simulink model "untitled"  (R2021a)
settings: Solver=VariableStepAuto  StartTime=0.0  StopTime=20000  RelTol=1e-3
values from neighbouring files (symbols this model uses):
  dtheta_GMO = sqrt(muy/r_GMO^3)    [Parameters.m]    (also in Spacecraft_Attitude_States.m)
  dtheta_LMO = sqrt(muy/r_LMO^3)    [Parameters.m]    (also in Spacecraft_Attitude_States.m)
  I = [10 0 0;0 5 0;0 0 7.5]    [Parameters.m]    (also in Spacecraft_Attitude_States.m)
  i0_GMO = 0    [Parameters.m]    (also in Spacecraft_Attitude_States.m)
  i0_LMO = pi/6    (= 0.523598775598)    [Parameters.m]    (also in Spacecraft_Attitude_States.m)
  K = 5    [Parameters.m]    (also in Spacecraft_Attitude_States.m)
  Omega0_GMO = 0    [Parameters.m]    (also in Spacecraft_Attitude_States.m)
  Omega0_LMO = pi/9    (= 0.349065850399)    [Parameters.m]    (also in Spacecraft_Attitude_States.m)
  P = 10*eye(3)    [Parameters.m]    (also in Spacecraft_Attitude_States.m)
  r_GMO = 20424.2*10^3    (= 20424200)    [Parameters.m]    (also in Spacecraft_Attitude_States.m = 20424.2)
  r_LMO = R + h    (= 3796190)    [Parameters.m]    (also in Spacecraft_Attitude_States.m = 3796.19)
  T1 = 800    [Parameters.m]
  T2 = 2500    [Parameters.m]
  theta0_GMO = 250*pi/180    (= 4.36332312999)    [Parameters.m]    (also in Spacecraft_Attitude_States.m)
  theta0_LMO = pi/3    (= 1.0471975512)    [Parameters.m]    (also in Spacecraft_Attitude_States.m)
libraries: sharedtransform x1
settings Model: Creator=VTX  LastModifiedBy=VTX

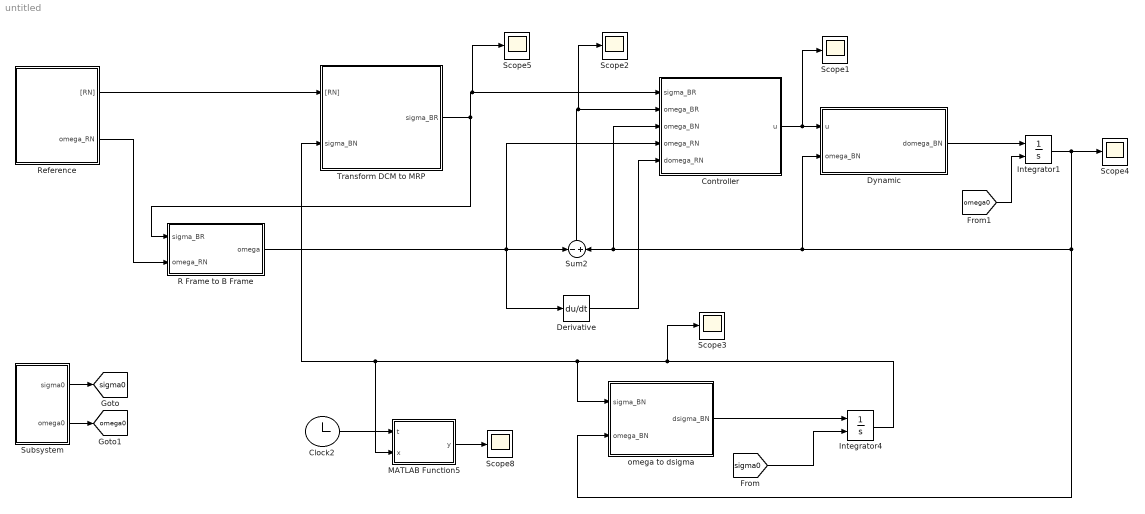
== system untitled ==
  Clock2 : Clock
  Controller : MATLAB Function  TreatAsAtomicUnit=on
  Derivative : Derivative
  Dynamic : MATLAB Function  TreatAsAtomicUnit=on
  Integrator1 : Integrator  InitialConditionSource=external  InitialCondition=[1;1.75;-2.2]*pi/180
  Integrator4 : Integrator  InitialConditionSource=external  InitialCondition=[0.3;-0.4;0.5]
  MATLAB Function5 : MATLAB Function  TreatAsAtomicUnit=on
  R Frame to B Frame : MATLAB Function  TreatAsAtomicUnit=on
  Reference : Subsystem
  Scope{1..5,8} (6 alike) : Scope
  Subsystem : Subsystem
  Sum2 : Sum  Inputs=-|+
  Transform DCM to MRP : Subsystem
  omega to dsigma : MATLAB Function  TreatAsAtomicUnit=on
  tag scope: omega0=global, sigma0=global
  wires:
  Integrator1/1 -> Dynamic/2(omega_BN), Controller/3(omega_BN), Sum2/2, omega to dsigma/2(omega_BN), Scope4/1
  Sum2/1 -> Scope2/1, Controller/2(omega_BR)
  [sigma0] -> Integrator4/2
  [omega0] -> Integrator1/2
  Derivative/1 -> Controller/5(domega_RN)
  Clock2/1 -> MATLAB Function5/1(t)
  Integrator4/1 -> Scope3/1, Transform DCM to MRP/2(sigma_BN), MATLAB Function5/2(x), omega to dsigma/1(sigma_BN)
  Subsystem/1(sigma0) -> [sigma0]
  Subsystem/2(omega0) -> [omega0]
  Dynamic/1(domega_BN) -> Integrator1/1
  Reference/1("[RN]") -> Transform DCM to MRP/1("[RN]")
  Transform DCM to MRP/1(sigma_BR) -> R Frame to B Frame/1(sigma_BR), Scope5/1, Controller/1(sigma_BR)
  R Frame to B Frame/1(omega) -> Sum2/1, Derivative/1, Controller/4(omega_RN)
  omega to dsigma/1(dsigma_BN) -> Integrator4/1
  Controller/1(u) -> Scope1/1, Dynamic/1(u)
  Reference/2(omega_RN) -> R Frame to B Frame/2(omega_RN)
  MATLAB Function5/1(y) -> Scope8/1

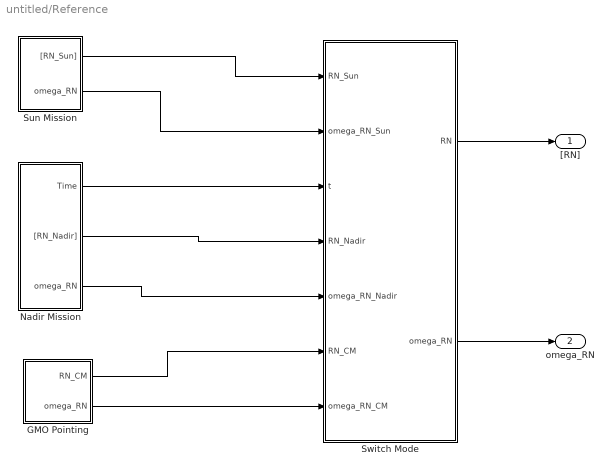
== system untitled/Reference ==
  GMO Pointing : Subsystem
  Nadir Mission : Subsystem
  Sun Mission : Subsystem
  Switch Mode : MATLAB Function  TreatAsAtomicUnit=on
  "[RN]" : Outport
  omega_RN : Outport  Port=2
  wires:
  Switch Mode/2(omega_RN) -> omega_RN/1
  Switch Mode/1(RN) -> "[RN]"/1
  Sun Mission/1("[RN_Sun]") -> Switch Mode/1(RN_Sun)
  Sun Mission/2(omega_RN) -> Switch Mode/2(omega_RN_Sun)
  Nadir Mission/1(Time) -> Switch Mode/3(t)
  Nadir Mission/2("[RN_Nadir]") -> Switch Mode/4(RN_Nadir)
  Nadir Mission/3(omega_RN) -> Switch Mode/5(omega_RN_Nadir)
  GMO Pointing/1(RN_CM) -> Switch Mode/6(RN_CM)
  GMO Pointing/2(omega_RN) -> Switch Mode/7(omega_RN_CM)

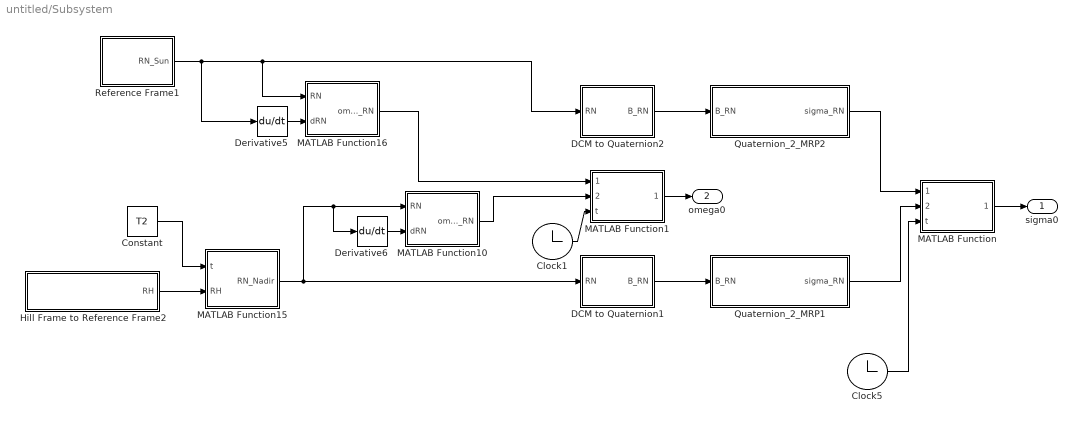
== system untitled/Subsystem ==
  Clock1 : Clock
  Clock5 : Clock
  Constant : Constant  Value=T2
  DCM to Quaternion1 : MATLAB Function  TreatAsAtomicUnit=on
  DCM to Quaternion2 : MATLAB Function  TreatAsAtomicUnit=on
  Derivative5 : Derivative
  Derivative6 : Derivative
  Hill Frame to Reference Frame2 : MATLAB Function  TreatAsAtomicUnit=on
  MATLAB Function : MATLAB Function  TreatAsAtomicUnit=on
  MATLAB Function1 : MATLAB Function  TreatAsAtomicUnit=on
  MATLAB Function10 : MATLAB Function  TreatAsAtomicUnit=on
  MATLAB Function15 : MATLAB Function  TreatAsAtomicUnit=on
  MATLAB Function16 : MATLAB Function  TreatAsAtomicUnit=on
  Quaternion_2_MRP1 : MATLAB Function  TreatAsAtomicUnit=on
  Quaternion_2_MRP2 : MATLAB Function  TreatAsAtomicUnit=on
  Reference Frame1 : MATLAB Function  TreatAsAtomicUnit=on
  sigma0 : Outport
  omega0 : Outport  Port=2
  wires:
  MATLAB Function15/1(RN_Nadir) -> DCM to Quaternion1/1(RN), Derivative6/1, MATLAB Function10/1(RN)
  Reference Frame1/1(RN_Sun) -> Derivative5/1, DCM to Quaternion2/1(RN), MATLAB Function16/1(RN)
  ? -> ?
  Hill Frame to Reference Frame2/1(RH) -> MATLAB Function15/2(RH)
  Derivative5/1 -> MATLAB Function16/2(dRN)
  MATLAB Function16/1(omega_RN) -> MATLAB Function1/1(omega_RN_Sun)
  Derivative6/1 -> MATLAB Function10/2(dRN)
  Constant/1 -> MATLAB Function15/1(t)
  DCM to Quaternion2/1(B_RN) -> Quaternion_2_MRP2/1(B_RN)
  DCM to Quaternion1/1(B_RN) -> Quaternion_2_MRP1/1(B_RN)
  Quaternion_2_MRP2/1(sigma_RN) -> MATLAB Function/1(sigma_RN_Sun)
  Quaternion_2_MRP1/1(sigma_RN) -> MATLAB Function/2(sigma_RN_Nadir)
  Clock5/1 -> MATLAB Function/3(t)
  MATLAB Function/1(sigma0) -> sigma0/1
  MATLAB Function10/1(omega_RN) -> MATLAB Function1/2(omega_RN_Nadir)
  Clock1/1 -> MATLAB Function1/3(t)
  MATLAB Function1/1(omega0) -> omega0/1

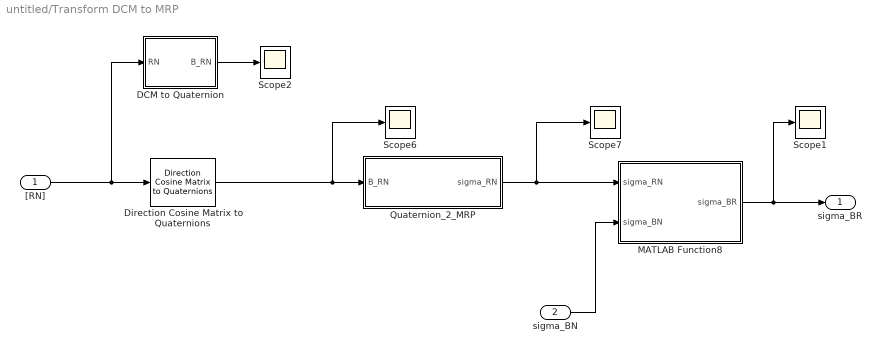
== system untitled/Transform DCM to MRP ==
  "[RN]" : Inport
  sigma_BN : Inport  Port=2
  DCM to Quaternion : MATLAB Function  TreatAsAtomicUnit=on
  Direction Cosine Matrix to Quaternions : sharedtransform/Direction Cosine Matrix  to Quaternions  aMode=0  action=None  tolerance=eps(2)
      settings: SourceProductBaseCode=AE,PW,DR,MT,UV,VE
  MATLAB Function8 : MATLAB Function  TreatAsAtomicUnit=on
  Quaternion_2_MRP : MATLAB Function  TreatAsAtomicUnit=on
  Scope{1..2,6..7} (4 alike) : Scope
  sigma_BR : Outport
  wires:
  Direction Cosine Matrix to Quaternions/1 -> Scope6/1, Quaternion_2_MRP/1(B_RN)
  Quaternion_2_MRP/1(sigma_RN) -> Scope7/1, MATLAB Function8/1(sigma_RN)
  sigma_BN/1 -> MATLAB Function8/2(sigma_BN)
  MATLAB Function8/1(sigma_BR) -> Scope1/1, sigma_BR/1
  "[RN]"/1 -> DCM to Quaternion/1(RN), Direction Cosine Matrix to Quaternions/1
  DCM to Quaternion/1(B_RN) -> Scope2/1

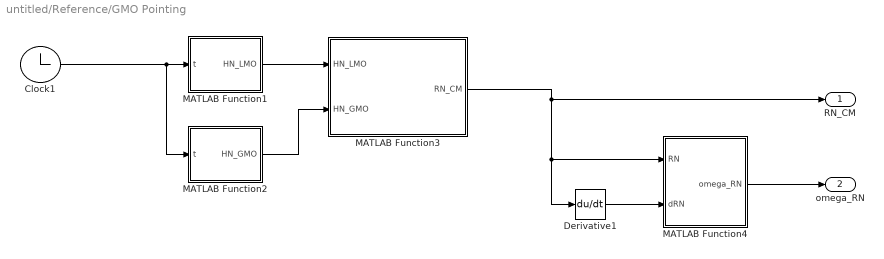
== system untitled/Reference/GMO Pointing ==
  Clock1 : Clock
  Derivative1 : Derivative
  MATLAB Function1 : MATLAB Function  TreatAsAtomicUnit=on
  MATLAB Function2 : MATLAB Function  TreatAsAtomicUnit=on
  MATLAB Function3 : MATLAB Function  TreatAsAtomicUnit=on
  MATLAB Function4 : MATLAB Function  TreatAsAtomicUnit=on
  RN_CM : Outport
  omega_RN : Outport  Port=2
  wires:
  Derivative1/1 -> MATLAB Function4/2(dRN)
  MATLAB Function1/1(HN_LMO) -> MATLAB Function3/1(HN_LMO)
  Clock1/1 -> MATLAB Function2/1(t), MATLAB Function1/1(t)
  MATLAB Function2/1(HN_GMO) -> MATLAB Function3/2(HN_GMO)
  MATLAB Function3/1(RN_CM) -> Derivative1/1, MATLAB Function4/1(RN), RN_CM/1
  MATLAB Function4/1(omega_RN) -> omega_RN/1

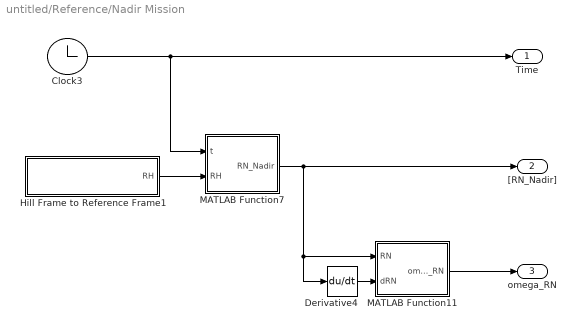
== system untitled/Reference/Nadir Mission ==
  Clock3 : Clock
  Derivative4 : Derivative
  Hill Frame to Reference Frame1 : MATLAB Function  TreatAsAtomicUnit=on
  MATLAB Function11 : MATLAB Function  TreatAsAtomicUnit=on
  MATLAB Function7 : MATLAB Function  TreatAsAtomicUnit=on
  Time : Outport
  "[RN_Nadir]" : Outport  Port=2
  omega_RN : Outport  Port=3
  wires:
  Clock3/1 -> Time/1, MATLAB Function7/1(t)
  MATLAB Function11/1(omega_RN) -> omega_RN/1
  MATLAB Function7/1(RN_Nadir) -> "[RN_Nadir]"/1, Derivative4/1, MATLAB Function11/1(RN)
  Hill Frame to Reference Frame1/1(RH) -> MATLAB Function7/2(RH)
  Derivative4/1 -> MATLAB Function11/2(dRN)

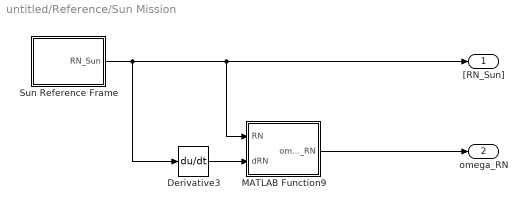
== system untitled/Reference/Sun Mission ==
  Derivative3 : Derivative
  MATLAB Function9 : MATLAB Function  TreatAsAtomicUnit=on
  Sun Reference Frame : MATLAB Function  TreatAsAtomicUnit=on
  "[RN_Sun]" : Outport
  omega_RN : Outport  Port=2
  wires:
  Derivative3/1 -> MATLAB Function9/2(dRN)
  Sun Reference Frame/1(RN_Sun) -> Derivative3/1, "[RN_Sun]"/1, MATLAB Function9/1(RN)
  MATLAB Function9/1(omega_RN) -> omega_RN/1

== matlab function untitled/Reference/GMO Pointing/MATLAB Function3 ==
  data: RN_CM output; HN_LMO input; HN_GMO input; r_LMO parameter; r_GMO parameter
function RN_CM = fcn(HN_LMO, HN_GMO,r_LMO, r_GMO)
    R_LMO = r_LMO*HN_LMO'*[1 0 0]';
    R_GMO = r_GMO*HN_GMO'*[1 0 0]';
    delta_R = R_GMO - R_LMO;
    
    r1 = delta_R/norm(delta_R);
    r2 = cross(delta_R,[0 0 1]')/norm(cross(delta_R,[0 0 1]'));
    r3 = cross(r1,r2);
    
    RN_CM = [r1 r2 r3]';
end

== matlab function untitled/Reference/GMO Pointing/MATLAB Function4 ==
  data: RN input; omega_RN output; dRN input
function omega_RN = fcn(RN,dRN)
    omega_RN_tidle = -dRN*RN';
    o1 = omega_RN_tidle(3,2);
    o2 = omega_RN_tidle(1,3);
    o3 = omega_RN_tidle(2,1);
    omega_RN = [o1 o2 o3]';
end

== matlab function untitled/MATLAB Function5 ==
  data: t input; y output; x input; T1 parameter
function y = fcn(t,x,T1)
    y = [0 0 0]';
    if t == T1
        y = x;
    end
end

== matlab function untitled/Subsystem/Hill Frame to Reference Frame2 ==
  data: RH output
function RH = fcn()
RH = [-1 0 0;0 1 0;0 0 -1];
end

== matlab function untitled/Subsystem/MATLAB Function10 ==
  data: RN input; omega_RN output; dRN input
function omega_RN = fcn(RN,dRN)
    omega_RN_tidle = -dRN*RN';
    o1 = omega_RN_tidle(3,2);
    o2 = omega_RN_tidle(1,3);
    o3 = omega_RN_tidle(2,1);
    omega_RN = [o1 o2 o3]';
end

== matlab function untitled/Subsystem/DCM to Quaternion2 ==
  data: RN input; B_RN output size=4
function B_RN = fcn(RN)
    trace = RN(1,1) + RN(2,2) + RN(3,3);
    beta0 = (0.25*(1 + trace));
    beta1 = (0.25*(1 + 2*RN(1,1) - trace));
    beta2 = (0.25*(1 + 2*RN(2,2) - trace));
    beta3 = (0.25*(1 + 2*RN(3,3) - trace));
    
    m = max([beta0 beta1 beta2 beta3]);

    B0 = 0; B1 = 0; B2 = 0; B3 = 0;
    
    if beta0 == m
        B0 = sqrt(beta0);
        B1 = (RN(2,3)-RN(3,2))/(4*B0);
        B2 = (RN(3,1)-RN(1,3))/(4*B0);
        B3 = (RN(1,2)-RN(2,1))/(4*B0);
    elseif beta1 == m
        B1 = sqrt(beta1);
        B0 = (RN(2,3)-RN(3,2))/(4*B1);
        B2 = (RN(1,2)+RN(2,1))/(4*B1);
        B3 = (RN(3,1)+RN(1,3))/(4*B1);
    elseif beta2 == m
        B2 = sqrt(beta2);
        B0 = (RN(3,1)-RN(1,3))/(4*B2);
        B1 = (RN(1,2)+RN(2,1))/(4*B2);
        B3 = (RN(2,3)+RN(3,2))/(4*B2);
    elseif beta3 == m
        B3 = sqrt(beta3);
        B0 = (RN(1,2)-RN(2,1))/(4*B3);
        B1 = (RN(3,1)+RN(1,3))/(4*B3);
        B2 = (RN(2,3)+RN(3,2))/(4*B3);
    end
    
    B_RN = [B0 B1 B2 B3]';
end

== matlab function untitled/Subsystem/Quaternion_2_MRP2 ==
  data: B_RN input; sigma_RN output
function sigma_RN  = fcn(B_RN)
    sigma1 = B_RN(2)/(1 + B_RN(1));
    sigma2 = B_RN(3)/(1 + B_RN(1));
    sigma3 = B_RN(4)/(1 + B_RN(1));
    
    sigma_RN = [sigma1 sigma2 sigma3]';

    if norm(sigma_RN) >= 1
        sigma1 = -B_RN(2)/(1 - B_RN(1));
        sigma2 = -B_RN(3)/(1 - B_RN(1));
        sigma3 = -B_RN(4)/(1 - B_RN(1));
    
        sigma_RN = [sigma1 sigma2 sigma3]';
    end   
end

== matlab function untitled/Subsystem/DCM to Quaternion1 ==
  data: RN input; B_RN output size=4
function B_RN = fcn(RN)
    trace = RN(1,1) + RN(2,2) + RN(3,3);
    beta0 = (0.25*(1 + trace));
    beta1 = (0.25*(1 + 2*RN(1,1) - trace));
    beta2 = (0.25*(1 + 2*RN(2,2) - trace));
    beta3 = (0.25*(1 + 2*RN(3,3) - trace));
    
    m = max([beta0 beta1 beta2 beta3]);

    B0 = 0; B1 = 0; B2 = 0; B3 = 0;
    
    if beta0 == m
        B0 = sqrt(beta0);
        B1 = (RN(2,3)-RN(3,2))/(4*B0);
        B2 = (RN(3,1)-RN(1,3))/(4*B0);
        B3 = (RN(1,2)-RN(2,1))/(4*B0);
    elseif beta1 == m
        B1 = sqrt(beta1);
        B0 = (RN(2,3)-RN(3,2))/(4*B1);
        B2 = (RN(1,2)+RN(2,1))/(4*B1);
        B3 = (RN(3,1)+RN(1,3))/(4*B1);
    elseif beta2 == m
        B2 = sqrt(beta2);
        B0 = (RN(3,1)-RN(1,3))/(4*B2);
        B1 = (RN(1,2)+RN(2,1))/(4*B2);
        B3 = (RN(2,3)+RN(3,2))/(4*B2);
    elseif beta3 == m
        B3 = sqrt(beta3);
        B0 = (RN(1,2)-RN(2,1))/(4*B3);
        B1 = (RN(3,1)+RN(1,3))/(4*B3);
        B2 = (RN(2,3)+RN(3,2))/(4*B3);
    end
    
    B_RN = [B0 B1 B2 B3]';
end

== matlab function untitled/Controller ==
  data: sigma_BR input; u output; omega_BR input; K parameter; P parameter; omega_BN input; omega_RN input; I parameter; domega_RN input
function u = fcn(sigma_BR,omega_BR,K,P,omega_BN,omega_RN, I,domega_RN)

    u = -K*sigma_BR - P*omega_BR;
    % u = -K*sigma_BR - P*omega_BR + I*(domega_RN - cross(omega_BN,omega_RN)) + cross(omega_BN,(I*omega_BN));
    
    u_max = 5;
    if abs(u) > u_max
        u = sign(u)*u_max;
    end
end

== matlab function untitled/Subsystem/MATLAB Function15 ==
  data: RN_Nadir output; t input; RH input; Omega0_LMO parameter; i0_LMO parameter; theta0_LMO parameter; dtheta_LMO parameter
function RN_Nadir  = fcn(t, RH,Omega0_LMO, i0_LMO, theta0_LMO, dtheta_LMO)
    %% Rotate about z axis
    Cz1 = [cos(Omega0_LMO) sin(Omega0_LMO) 0;-sin(Omega0_LMO) cos(Omega0_LMO) 0;0 0 1];

    %% Rotate about x axis
    Cx2 = [1 0 0;0 cos(i0_LMO) sin(i0_LMO);0 -sin(i0_LMO) cos(i0_LMO)];
    
    %% Rotate about z axis
    Cz3 = [cos(theta0_LMO + dtheta_LMO*t) sin(theta0_LMO + dtheta_LMO*t) 0;-sin(theta0_LMO + dtheta_LMO*t) cos(theta0_LMO + dtheta_LMO*t) 0;0 0 1];

    %% DCM from Inertial Frame to Hill Frame
    HN = Cz3*Cx2*Cz1;
    
    %% DCm from Inertial Frame to Reference Frame
    RN_Nadir = RH*HN;
end

== matlab function untitled/Subsystem/MATLAB Function16 ==
  data: RN input; omega_RN output; dRN input
function omega_RN = fcn(RN,dRN)
    omega_RN_tidle = -dRN*RN';
    o1 = omega_RN_tidle(3,2);
    o2 = omega_RN_tidle(1,3);
    o3 = omega_RN_tidle(2,1);
    omega_RN = [o1 o2 o3]';
end

== matlab function untitled/Subsystem/Quaternion_2_MRP1 ==
  data: B_RN input; sigma_RN output
function sigma_RN  = fcn(B_RN)
    sigma1 = B_RN(2)/(1 + B_RN(1));
    sigma2 = B_RN(3)/(1 + B_RN(1));
    sigma3 = B_RN(4)/(1 + B_RN(1));
    
    sigma_RN = [sigma1 sigma2 sigma3]';

    if norm(sigma_RN) >= 1
        sigma1 = -B_RN(2)/(1 - B_RN(1));
        sigma2 = -B_RN(3)/(1 - B_RN(1));
        sigma3 = -B_RN(4)/(1 - B_RN(1));
    
        sigma_RN = [sigma1 sigma2 sigma3]';
    end   
end

== matlab function untitled/Subsystem/Reference Frame1 ==
  data: RN_Sun output
function RN_Sun = fcn()
    RN_Sun = [-1 0 0;0 0 1;0 1 0];
end

== matlab function untitled/Subsystem/MATLAB Function ==
  data: sigma_RN_Sun input; sigma0 output; sigma_RN_Nadir input; t input; T1 parameter; T2 parameter
function sigma0 = fcn(sigma_RN_Sun,sigma_RN_Nadir,t,T1, T2)
    if t < T1
        sigma0 = [0.3;-0.4;0.5];
    elseif (t >= T1) && (t < T2)
        sigma0 = sigma_RN_Sun;
    else
        sigma0 = sigma_RN_Nadir;
    end
end

== matlab function untitled/Transform DCM to MRP/MATLAB Function8 ==
  data: sigma_BR output; sigma_RN input; sigma_BN input
function sigma_BR = fcn(sigma_RN, sigma_BN)
    sigma_BR = ((1 - norm(sigma_RN)^2)*sigma_BN - (1 - norm(sigma_BN)^2)*sigma_RN + 2*cross(sigma_BN,sigma_RN))/(1 + norm(sigma_RN)^2*norm(sigma_BN)^2 + 2*dot(sigma_RN,sigma_BN));
end

== matlab function untitled/Reference/Sun Mission/MATLAB Function9 ==
  data: RN input; omega_RN output; dRN input
function omega_RN = fcn(RN,dRN)
    omega_RN_tidle = -dRN*RN';
    o1 = omega_RN_tidle(3,2);
    o2 = omega_RN_tidle(1,3);
    o3 = omega_RN_tidle(2,1);
    omega_RN = [o1 o2 o3]';
end

== matlab function untitled/Transform DCM to MRP/Quaternion_2_MRP ==
  data: B_RN input; sigma_RN output
function sigma_RN  = fcn(B_RN)
    sigma1 = B_RN(2)/(1 + B_RN(1));
    sigma2 = B_RN(3)/(1 + B_RN(1));
    sigma3 = B_RN(4)/(1 + B_RN(1));
    
    sigma_RN = [sigma1 sigma2 sigma3]';

    if norm(sigma_RN) >= 1
        sigma1 = -B_RN(2)/(1 - B_RN(1));
        sigma2 = -B_RN(3)/(1 - B_RN(1));
        sigma3 = -B_RN(4)/(1 - B_RN(1));
    
        sigma_RN = [sigma1 sigma2 sigma3]';
    end   
end

== matlab function untitled/Reference/Sun Mission/Sun Reference Frame ==
  data: RN_Sun output
function RN_Sun = fcn()
    RN_Sun = [-1 0 0;0 0 1;0 1 0];
end

== matlab function untitled/Reference/Switch Mode ==
  data: RN_Sun input; omega_RN_Sun input; t input; RN_Nadir input; omega_RN_Nadir input; RN output; omega_RN output; RN_CM input; omega_RN_CM input; T1 parameter; T2 parameter
function [RN,omega_RN] = fcn(RN_Sun,omega_RN_Sun, t, RN_Nadir,omega_RN_Nadir,RN_CM,omega_RN_CM,T1, T2)
    RN = RN_Sun;
    omega_RN = omega_RN_Sun;
    if t > T1 && t <= T2
        RN = RN_Nadir;
        omega_RN = omega_RN_Nadir;
    elseif t > T2
        RN = RN_CM;
        omega_RN = omega_RN_CM;
    end
end

== matlab function untitled/omega to dsigma ==
  data: sigma_BN input; dsigma_BN output size=3; omega_BN input
function dsigma_BN = fcn(sigma_BN,omega_BN)
   sigma_tilde = [0 -sigma_BN(3) sigma_BN(2);sigma_BN(3) 0 -sigma_BN(1);-sigma_BN(2) sigma_BN(1) 0];
   dsigma_BN = 1/4*((1 - dot(sigma_BN,sigma_BN))*eye(3) + 2*sigma_tilde + 2*sigma_BN*sigma_BN')*omega_BN;
end

== matlab function untitled/Subsystem/MATLAB Function1 ==
  data: omega_RN_Sun input; omega0 output; omega_RN_Nadir input; t input; T1 parameter; T2 parameter
function omega0 = fcn(omega_RN_Sun,omega_RN_Nadir,t,T1, T2)
    if t < T1
        omega0 = [1;1.75;-2.2]*pi/180;
    elseif (t >= T1) && (t < T2)
        omega0 = omega_RN_Sun;
    else
        omega0 = omega_RN_Nadir;
    end
end

== matlab function untitled/Transform DCM to MRP/DCM to Quaternion ==
  data: RN input; B_RN output size=4
function B_RN = fcn(RN)
    trace = RN(1,1) + RN(2,2) + RN(3,3);
    beta0 = (0.25*(1 + trace));
    beta1 = (0.25*(1 + 2*RN(1,1) - trace));
    beta2 = (0.25*(1 + 2*RN(2,2) - trace));
    beta3 = (0.25*(1 + 2*RN(3,3) - trace));
    
    m = max([beta0 beta1 beta2 beta3]);

    B0 = 0; B1 = 0; B2 = 0; B3 = 0;
    
    if beta0 == m
        B0 = sqrt(beta0);
        B1 = (RN(2,3)-RN(3,2))/(4*B0);
        B2 = (RN(3,1)-RN(1,3))/(4*B0);
        B3 = (RN(1,2)-RN(2,1))/(4*B0);
    elseif beta1 == m
        B1 = sqrt(beta1);
        B0 = (RN(2,3)-RN(3,2))/(4*B1);
        B2 = (RN(1,2)+RN(2,1))/(4*B1);
        B3 = (RN(3,1)+RN(1,3))/(4*B1);
    elseif beta2 == m
        B2 = sqrt(beta2);
        B0 = (RN(3,1)-RN(1,3))/(4*B2);
        B1 = (RN(1,2)+RN(2,1))/(4*B2);
        B3 = (RN(2,3)+RN(3,2))/(4*B2);
    elseif beta3 == m
        B3 = sqrt(beta3);
        B0 = (RN(1,2)-RN(2,1))/(4*B3);
        B1 = (RN(3,1)+RN(1,3))/(4*B3);
        B2 = (RN(2,3)+RN(3,2))/(4*B3);
    end
    
    B_RN = [B0 B1 B2 B3]';
end

== matlab function untitled/Dynamic ==
  data: u input; domega_BN output size=3; omega_BN input; I parameter
function domega_BN = fcn(u,omega_BN, I)
    domega_BN = inv(I)*(cross(omega_BN,(I*omega_BN)) + u);
end

== matlab function untitled/Reference/Nadir Mission/Hill Frame to Reference Frame1 ==
  data: RH output
function RH = fcn()
RH = [-1 0 0;0 1 0;0 0 -1];
end

== matlab function untitled/R Frame to B Frame ==
  data: omega output; sigma_BR input; omega_RN input
function omega = fcn(sigma_BR, omega_RN)
    %% This function returns a DCM that is transformed from MRP
    s1 = sigma_BR(1);
    s2 = sigma_BR(2);
    s3 = sigma_BR(3);
    
    sigma_cross = [0 -s3 s2;s3 0 -s1;-s2 s1 0];
    
    DCM = eye(3) + (8*sigma_cross*sigma_cross - 4*(1 - dot(sigma_BR,sigma_BR))*sigma_cross)/(1 + dot(sigma_BR,sigma_BR))^2;
    
    omega  = DCM*omega_RN;
end

== matlab function untitled/Reference/Nadir Mission/MATLAB Function11 ==
  data: RN input; omega_RN output; dRN input
function omega_RN = fcn(RN,dRN)
    omega_RN_tidle = -dRN*RN';
    o1 = omega_RN_tidle(3,2);
    o2 = omega_RN_tidle(1,3);
    o3 = omega_RN_tidle(2,1);
    omega_RN = [o1 o2 o3]';
end

== matlab function untitled/Reference/GMO Pointing/MATLAB Function1 ==
  data: t input; HN_LMO output; Omega0_LMO parameter; i0_LMO parameter; theta0_LMO parameter; dtheta_LMO parameter
function HN_LMO  = fcn(t,Omega0_LMO, i0_LMO, theta0_LMO, dtheta_LMO)
    %% Rotate about z axis
    Cz1 = [cos(Omega0_LMO) sin(Omega0_LMO) 0;-sin(Omega0_LMO) cos(Omega0_LMO) 0;0 0 1];

    %% Rotate about x axis
    Cx2 = [1 0 0;0 cos(i0_LMO) sin(i0_LMO);0 -sin(i0_LMO) cos(i0_LMO)];
    
    %% Rotate about z axis
    Cz3 = [cos(theta0_LMO + dtheta_LMO*t) sin(theta0_LMO + dtheta_LMO*t) 0;-sin(theta0_LMO + dtheta_LMO*t) cos(theta0_LMO + dtheta_LMO*t) 0;0 0 1];

    %% DCM from Inertial Frame to Hill Frame
    HN_LMO = Cz3*Cx2*Cz1;
end

== matlab function untitled/Reference/Nadir Mission/MATLAB Function7 ==
  data: RN_Nadir output; t input; RH input; Omega0_LMO parameter; i0_LMO parameter; theta0_LMO parameter; dtheta_LMO parameter
function RN_Nadir  = fcn(t, RH,Omega0_LMO, i0_LMO, theta0_LMO, dtheta_LMO)
    %% Rotate about z axis
    Cz1 = [cos(Omega0_LMO) sin(Omega0_LMO) 0;-sin(Omega0_LMO) cos(Omega0_LMO) 0;0 0 1];

    %% Rotate about x axis
    Cx2 = [1 0 0;0 cos(i0_LMO) sin(i0_LMO);0 -sin(i0_LMO) cos(i0_LMO)];
    
    %% Rotate about z axis
    Cz3 = [cos(theta0_LMO + dtheta_LMO*t) sin(theta0_LMO + dtheta_LMO*t) 0;-sin(theta0_LMO + dtheta_LMO*t) cos(theta0_LMO + dtheta_LMO*t) 0;0 0 1];

    %% DCM from Inertial Frame to Hill Frame
    HN = Cz3*Cx2*Cz1;
    
    %% DCm from Inertial Frame to Reference Frame
    RN_Nadir = RH*HN;
end

== matlab function untitled/Reference/GMO Pointing/MATLAB Function2 ==
  data: t input; HN_GMO output; Omega0_GMO parameter; i0_GMO parameter; theta0_GMO parameter; dtheta_GMO parameter
function HN_GMO  = fcn(t,Omega0_GMO, i0_GMO, theta0_GMO, dtheta_GMO)
    %% Rotate about z axis
    Cz1 = [cos(Omega0_GMO) sin(Omega0_GMO) 0;-sin(Omega0_GMO) cos(Omega0_GMO) 0;0 0 1];

    %% Rotate about x axis
    Cx2 = [1 0 0;0 cos(i0_GMO) sin(i0_GMO);0 -sin(i0_GMO) cos(i0_GMO)];
    
    %% Rotate about z axis
    Cz3 = [cos(theta0_GMO + dtheta_GMO*t) sin(theta0_GMO + dtheta_GMO*t) 0;-sin(theta0_GMO + dtheta_GMO*t) cos(theta0_GMO + dtheta_GMO*t) 0;0 0 1];

    %% DCM from Inertial Frame to Hill Frame
    HN_GMO = Cz3*Cx2*Cz1;
end
